simulink model "Wing_bending_mode_observer_sim_example"  (R2018b)
settings: Solver=ode45  StartTime=0.0  StopTime=10  FixedStep=sample_time  RelTol=1e-3
undefined symbols (not defined in the file or in its folder): DiscIntNeverNeededParam, imu_acc_bias, imu_acc_bias_gain, imu_acc_noise_gain, imu_gyro_bias, imu_gyro_bias_gain, imu_gyro_noise_gain, Phi_roll_sim, Phi_z_sim, structure, structure_red, structureGetNodeCg, structureGetNodeMass, structureGetTotalInertia, structureGetTotalMass, WBMO, WBMO_notune
libraries: simulink x3, filters_lib x2, flexibleBody_lib x1, everscale_lib x1
settings Model: Creator=milic  LastModifiedBy=yannic

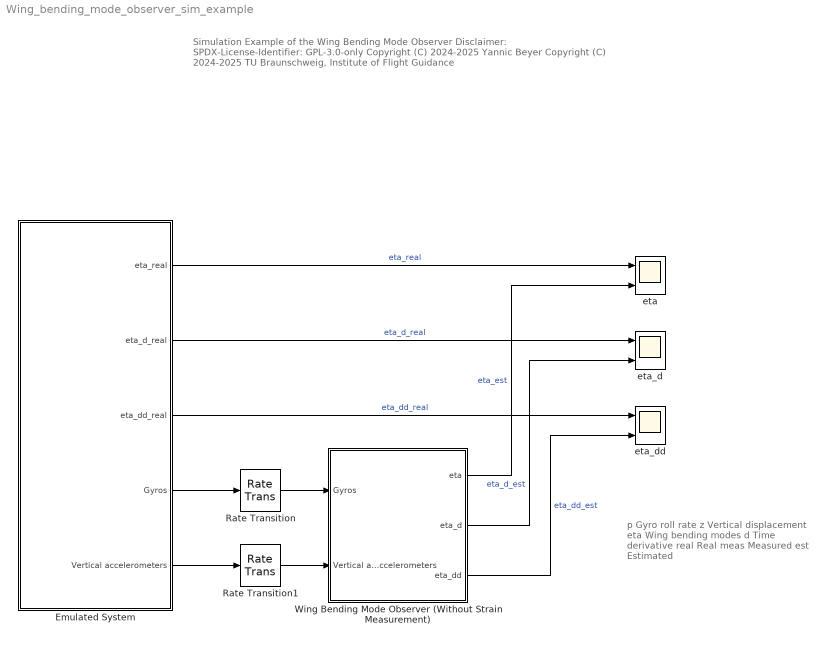
== system Wing_bending_mode_observer_sim_example ==
  note: p
      | Gyro roll rate
      |
      | z
      | Vertical displacement
      |
      | eta
      | Wing bending modes
      |
      | d
      | Time derivative
      |
      | real
      | Real
      |
      | meas
      | Measured
      |
      | est
      | Estimated
  note: Simulation Example of the Wing Bending Mode Observer
      |
      | Disclaimer:
      | SPDX-License-Identifier: GPL-3.0-only
      |
      | Copyright (C) 2024-2025 Yannic Beyer
      | Copyright (C) 2024-2025 TU Braunschweig, Institute of Flight Guidance
  Emulated System : Subsystem
  Rate Transition : RateTransition
  Rate Transition1 : RateTransition
  Wing Bending Mode Observer (Without Strain Measurement) : Subsystem
  eta : Scope  NumInputPorts=2
  eta_d : Scope  NumInputPorts=2
  eta_dd : Scope  NumInputPorts=2
  wires:
  Wing Bending Mode Observer (Without Strain Measurement)/3(eta_dd) -> eta_dd/2  "eta_dd_est"
  Wing Bending Mode Observer (Without Strain Measurement)/1(eta) -> eta/2  "eta_est"
  Wing Bending Mode Observer (Without Strain Measurement)/2(eta_d) -> eta_d/2  "eta_d_est"
  Emulated System/1(eta_real) -> eta/1  "eta_real"
  Emulated System/4(Gyros) -> Rate Transition/1
  Emulated System/2(eta_d_real) -> eta_d/1  "eta_d_real"
  Emulated System/5(Vertical accelerometers) -> Rate Transition1/1
  Emulated System/3(eta_dd_real) -> eta_dd/1  "eta_dd_real"
  Rate Transition/1 -> Wing Bending Mode Observer (Without Strain Measurement)/1(Gyros)
  Rate Transition1/1 -> Wing Bending Mode Observer (Without Strain Measurement)/2(Vertical accelerometers)

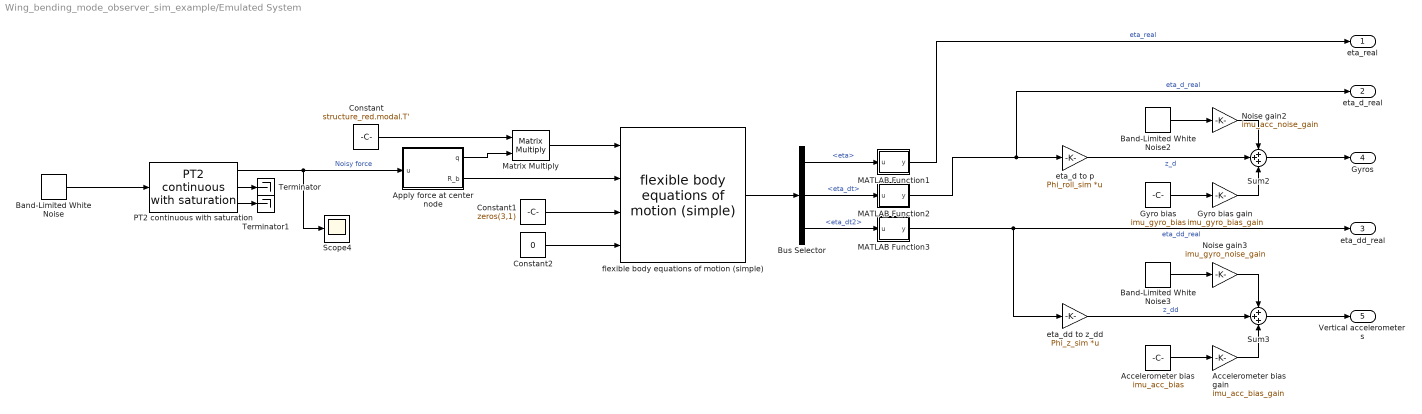
== system Wing_bending_mode_observer_sim_example/Emulated System ==
  Accelerometer bias : Constant  Value=imu_acc_bias
  Accelerometer bias gain : Gain  Gain=imu_acc_bias_gain
  Apply force at center node : MATLAB Function  TreatAsAtomicUnit=on
  Band-Limited White Noise : simulink/Sources/Band-Limited White Noise  Cov=2  Ts=WBMO_notune.sample_time  seed=[23341]
  Band-Limited White Noise2 : simulink/Sources/Band-Limited White Noise  Cov=[0.0001]  Ts=WBMO_notune.sample_time  seed=1:size(Phi_z_sim,1)
  Band-Limited White Noise3 : simulink/Sources/Band-Limited White Noise  Cov=[0.0001]  Ts=WBMO_notune.sample_time  seed=1:size(Phi_z_sim,1)
  Bus Selector : BusSelector  OutputSignals=eta,eta_dt,eta_dt2
  Constant : Constant  Value=structure_red.modal.T'
  Constant1 : Constant  Value=zeros(3,1)
  Constant2 : Constant  Value=0
  Gyro bias : Constant  Value=imu_gyro_bias
  Gyro bias gain : Gain  Gain=imu_gyro_bias_gain
  MATLAB Function1 : MATLAB Function  TreatAsAtomicUnit=on
  MATLAB Function2 : MATLAB Function  TreatAsAtomicUnit=on
  MATLAB Function3 : MATLAB Function  TreatAsAtomicUnit=on
  Matrix Multiply : Product  Multiplication=Matrix(*)
  Noise gain2 : Gain  Gain=imu_acc_noise_gain
  Noise gain3 : Gain  Gain=imu_gyro_noise_gain
  PT2 continuous with saturation : filters_lib/PT2 continuous with saturation  omega=150  d=0.7  x_dt2_max=inf  x_dt2_min=-inf  x_dt_max=inf  x_dt_min=-inf  x_max=inf  x_min=-inf  x_init=0  x_dt_init=0
      settings: SourceProductName=LADAC
  Scope4 : Scope
  Sum2 : Sum  Inputs=+++
  Sum3 : Sum  Inputs=+++
  Terminator : Terminator
  Terminator1 : Terminator
  eta_d to p : Gain  Gain=Phi_roll_sim  Multiplication=Matrix(K*u)
  eta_dd to z_dd : Gain  Gain=Phi_z_sim  Multiplication=Matrix(K*u)
  flexible body equations of motion (simple) : flexibleBody_lib/flexible body equations of motion (simple)  structure_red=structure_red  m=structureGetTotalMass(structure)  I_b=structureGetTotalInertia(structure)  m_nodes=structureGetNodeMass(structure,1:length(structure.xyz))  cg_nodes=structureGetNodeCg(structure,1:length(structure.xyz))  structure_vel_0=zeros(size(structure_red.K,2)-6,1)  structure_pos_0=zeros(size(structure_red.K,2)-6,1)
      settings: SourceProductName=LADAC
  eta_real : Outport
  eta_d_real : Outport  Port=2
  eta_dd_real : Outport  Port=3
  Gyros : Outport  Port=4
  Vertical accelerometers : Outport  Port=5
  wires:
  Constant/1 -> Matrix Multiply/1
  eta_dd to z_dd/1 -> Sum3/2  "z_dd"
  PT2 continuous with saturation/3 -> Terminator1/1
  Accelerometer bias/1 -> Accelerometer bias gain/1
  Matrix Multiply/1 -> flexible body equations of motion (simple)/1
  Accelerometer bias gain/1 -> Sum3/3
  MATLAB Function2/1(y) -> eta_d to p/1, eta_d_real/1  "eta_d_real"
  Sum2/1 -> Gyros/1
  Band-Limited White Noise3/1 -> Noise gain3/1
  Noise gain3/1 -> Sum3/1
  MATLAB Function1/1(y) -> eta_real/1  "eta_real"
  MATLAB Function3/1(y) -> eta_dd_real/1, eta_dd to z_dd/1  "eta_dd_real"
  Bus Selector/2 -> MATLAB Function2/1(u)  "<eta_dt>"
  Constant1/1 -> flexible body equations of motion (simple)/3
  Sum3/1 -> Vertical accelerometers/1
  Band-Limited White Noise2/1 -> Noise gain2/1
  PT2 continuous with saturation/2 -> Terminator/1
  Apply force at center node/2(R_b) -> flexible body equations of motion (simple)/2
  Constant2/1 -> flexible body equations of motion (simple)/4
  flexible body equations of motion (simple)/1 -> Bus Selector/1
  PT2 continuous with saturation/1 -> Scope4/1, Apply force at center node/1(u)  "Noisy force"
  Band-Limited White Noise/1 -> PT2 continuous with saturation/1
  eta_d to p/1 -> Sum2/2  "z_d"
  Apply force at center node/1(q) -> Matrix Multiply/2
  Bus Selector/1 -> MATLAB Function1/1(u)  "<eta>"
  Bus Selector/3 -> MATLAB Function3/1(u)  "<eta_dt2>"
  Noise gain2/1 -> Sum2/1
  Gyro bias/1 -> Gyro bias gain/1
  Gyro bias gain/1 -> Sum2/3

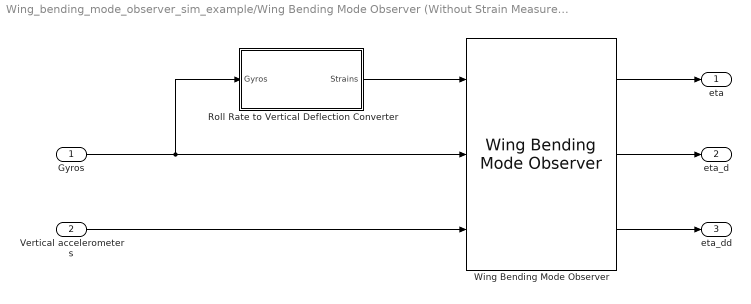
== system Wing_bending_mode_observer_sim_example/Wing Bending Mode Observer (Without Strain Measurement) ==
  Gyros : Inport  SampleTime=WBMO_notune.sample_time
  Vertical accelerometers : Inport  Port=2  SampleTime=WBMO_notune.sample_time
  Roll Rate to Vertical Deflection Converter : Subsystem
  Wing Bending Mode Observer : everscale_lib/Wing Bending Mode Observer  wbmo=WBMO  wbmo_notune=WBMO_notune
  eta : Outport
  eta_d : Outport  Port=2
  eta_dd : Outport  Port=3
  wires:
  Vertical accelerometers/1 -> Wing Bending Mode Observer/3
  Wing Bending Mode Observer/1 -> eta/1
  Wing Bending Mode Observer/2 -> eta_d/1
  Wing Bending Mode Observer/3 -> eta_dd/1
  Gyros/1 -> Wing Bending Mode Observer/2, Roll Rate to Vertical Deflection Converter/1(Gyros)
  Roll Rate to Vertical Deflection Converter/1(Strains) -> Wing Bending Mode Observer/1

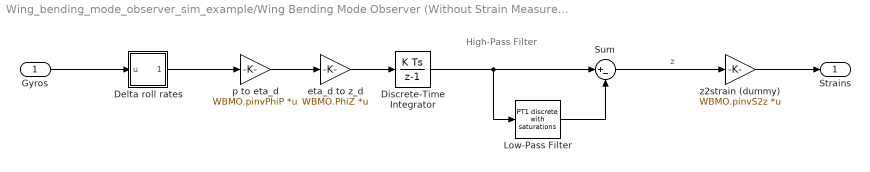
== system Wing_bending_mode_observer_sim_example/Wing Bending Mode Observer (Without Strain Measurement)/Roll Rate to Vertical Deflection Converter ==
  note: High-Pass Filter
  Gyros : Inport
  Delta roll rates : MATLAB Function  TreatAsAtomicUnit=on
  Discrete-Time Integrator : DiscreteIntegrator  SampleTime=-1  ICPrevOutput=DiscIntNeverNeededParam  ICPrevScaledInput=DiscIntNeverNeededParam
  Low-Pass Filter : filters_lib/PT1 discrete with saturations  param_src=internal  T=WBMO.T  x_max=inf  x_min=-inf  x_dt_max=inf  x_dt_min=-inf  y_0_src=internal  x_init=0  is_y_dt_checked=off  is_external_reset_checked=off  mask_expr_handling_config=default
      settings: SourceProductName=LADAC
  Sum : Sum  Inputs=|+-
  eta_d to z_d : Gain  Gain=WBMO.PhiZ  Multiplication=Matrix(K*u)
  p to eta_d : Gain  Gain=WBMO.pinvPhiP  Multiplication=Matrix(K*u)
  z2strain (dummy) : Gain  Gain=WBMO.pinvS2z  Multiplication=Matrix(K*u)
  Strains : Outport
  wires:
  Sum/1 -> z2strain (dummy)/1  "z"
  Low-Pass Filter/1 -> Sum/2
  eta_d to z_d/1 -> Discrete-Time Integrator/1
  Gyros/1 -> Delta roll rates/1(u)
  Discrete-Time Integrator/1 -> Low-Pass Filter/1, Sum/1
  p to eta_d/1 -> eta_d to z_d/1
  z2strain (dummy)/1 -> Strains/1
  Delta roll rates/1(Delta_u) -> p to eta_d/1

== matlab function Wing_bending_mode_observer_sim_example/Emulated System/Apply force at center node ==
  data: u input; q output; R_b output; num_nodes parameter
function [q,R_b] = fcn(u,num_nodes)
q = zeros(6*num_nodes,1);
q((num_nodes/2-0.5)*6+3) = u;
R_b = zeros(3,1);
R_b(3) = u;
end

== matlab function Wing_bending_mode_observer_sim_example/Emulated System/MATLAB Function1 ==
  data: u input; y output
function y = fcn(u)
y = u(7:end);
end

== matlab function Wing_bending_mode_observer_sim_example/Emulated System/MATLAB Function2 ==
  data: u input; y output
function y = fcn(u)
y = u(7:end);
end

== matlab function Wing_bending_mode_observer_sim_example/Emulated System/MATLAB Function3 ==
  data: u input; y output
function y = fcn(u)
y = u(7:end);
end

== matlab function Wing_bending_mode_observer_sim_example/Wing Bending Mode Observer (Without Strain Measurement)/Roll Rate to Vertical Deflection Converter/Delta roll rates ==
  data: u input; Delta_u output
function Delta_u = fcn(u)
Delta_u = zeros(length(u)-1,1);
u_center = u(end/2+0.5);
Delta_u(1:end/2) = u(1:end/2-0.5) - u_center;
Delta_u(end/2+1:end) = u(end/2+1.5:end) - u_center;
end
